simulink model "Passive_Road_profile_1"  (R2017b)
settings: Solver=VariableStepAuto  StartTime=0.0  StopTime=40  RelTol=1e-3
undefined symbols (not defined in the file): sigbuilder_block
settings Model: Creator=LENOVO  LastModifiedBy=LENOVO

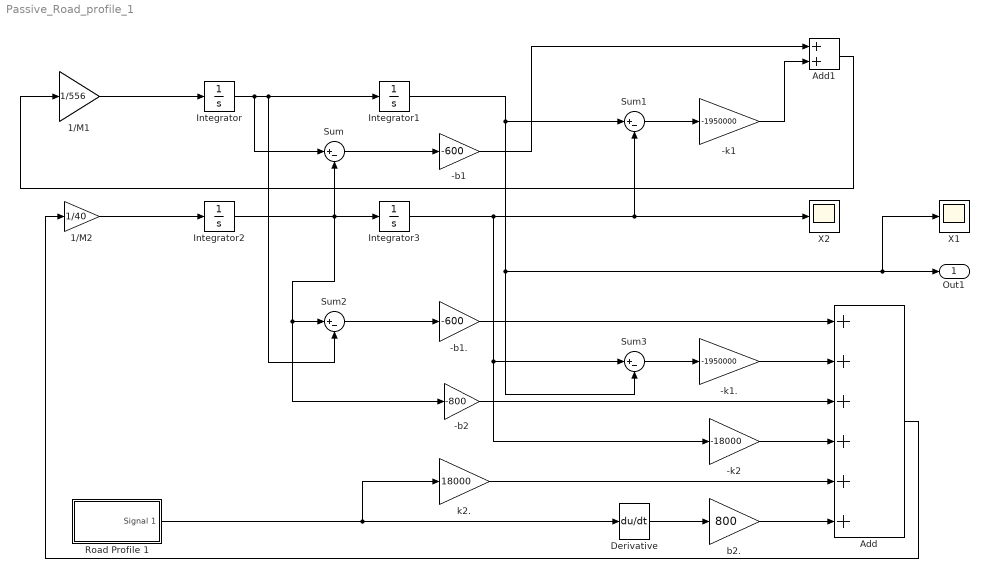
== system Passive_Road_profile_1 ==
  -b1 : Gain  Gain=-600
  -b1. : Gain  Gain=-600
  -b2 : Gain  Gain=-800
  -k1 : Gain  Gain=-1950000
  -k1. : Gain  Gain=-1950000
  -k2 : Gain  Gain=-18000
  1/M1 : Gain  Gain=1/556
  1/M2 : Gain  Gain=1/40
  Add : Sum  Inputs=++++++
  Add1 : Sum
  Derivative : Derivative
  Integrator{,1..3} (4 alike) : Integrator
  Road Profile 1 : Subsystem  Tag=STV Subsys  LoadFcn=sigbuilder_block('load');  StartFcn=sigbuilder_block('start');  StopFcn=sigbuilder_block('stop');  ClipboardFcn=sigbuilder_block('clipboard');  mask(Sigbuilder block){tuvar=[0:10]}
      mask help: Simulink:masks:SigbuilderBlock_MD
      mask init:
      | if ~strcmp(get_param(bdroot(gcbh),'SimulationStatus'),'stopped') tuvar = sigbuilder_block('maskInit'); end
      settings: CopyFcn=sigbuilder_block('copy');  DeleteFcn=sigbuilder_block('delete');  ModelCloseFcn=sigbuilder_block('modelClose');  PreSaveFcn=sigbuilder_block('preSave');  PauseFcn=sigbuilder_block('pause');  ContinueFcn=sigbuilder_block('continue');  NameChangeFcn=sigbuilder_block('namechange');  OpenFcn=sigbuilder_block('open',[6 0 1012.5 477.75 ]);  CloseFcn=sigbuilder_block('close');
      mask Display: plot(0, 0, 100, 100,[2, 2, 32, 32, 2], [68, 8, 8, 68, 68],[32, 2], [38, 38], [32, 19, 2],[53, 60, 44], [32, 17, 17, 2],[16, 16, 31, 31]);txt = getActiveGroup(gcbh);text(2, 100, txt,'verticalAlignment', 'top');
  Sum{,1..3} (4 alike) : Sum  Inputs=|+-
  X1 : Scope
  X2 : Scope
  b2. : Gain  Gain=800
  k2. : Gain  Gain=18000
  Out1 : Outport
  wires:
  1/M2/1 -> Integrator2/1
  Integrator3/1 -> Sum3/1, -k2/1, Sum1/2, X2/1
  Integrator2/1 -> Sum2/1, -b2/1, Sum/2, Integrator3/1
  Sum2/1 -> -b1./1
  Sum/1 -> -b1/1
  Integrator/1 -> Sum/1, Sum2/2, Integrator1/1
  -b1/1 -> Add1/1
  Sum3/1 -> -k1./1
  k2./1 -> Add/5
  Add/1 -> 1/M2/1
  -k1/1 -> Add1/2
  -k1./1 -> Add/2
  -k2/1 -> Add/4
  Derivative/1 -> b2./1
  -b2/1 -> Add/3
  -b1./1 -> Add/1
  Integrator1/1 -> Sum1/1, X1/1, Out1/1, Sum3/2
  Sum1/1 -> -k1/1
  Road Profile 1/1(Signal 1) -> Derivative/1, k2./1
  b2./1 -> Add/6
  1/M1/1 -> Integrator/1
  Add1/1 -> 1/M1/1

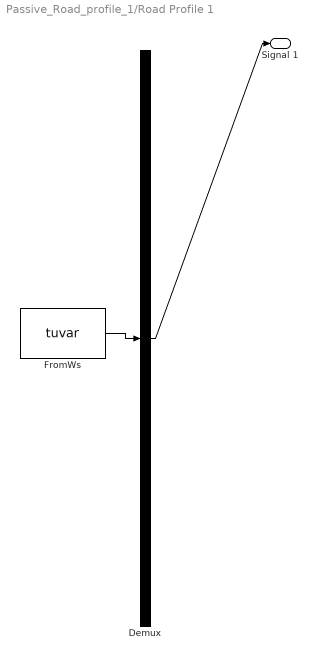
== system Passive_Road_profile_1/Road Profile 1 ==
  Demux : Demux  Tag=STV Demux  Outputs=1
  FromWs : FromWorkspace  Tag=STV FromWs  VariableName=tuvar  SampleTime=0
      SigBuilderData=|
      | common.afterFinalStr = 'Extrapolate'
      | common.sampleTime = 0
      | dataSet.timeRange = [0 40]
      | dataSet.name = 'Group 1'
      | sbobj.Groups.Name = 'Group 1'
      | sbobj.Groups.Signals.Name = 'Signal 1'
      | sbobj.Groups.Signals.XData = [0 2 3 4 5 7 10 11 12 13 14 15 16 17 18 19 20 21 22 23 24 25 26 27 28 29 30 31 32 33 34 35 36 37 38 40]
      | sbobj.Groups.Signals.YData = [0 0 0 0 0 0.1 0 0 0 0 0 0 0 0 0 0 0 0 0 0 0 0 0 0 0 0 0 0 0 0 0 0 0 0 0 0]
      | sbobj.Groups.TimeRange = [0 40]
  Signal 1 : Outport  Tag=STV Outport
  wires:
  FromWs/1 -> Demux/1
  Demux/1 -> Signal 1/1
